simulink model "LCL_singlephase_ESO_UIO"  (R2023b)
settings: Solver=FixedStepAuto  StartTime=0.0  StopTime=0.4  FixedStep=step_time  RelTol=1e-3  EnableMultiTasking=on
values from neighbouring files (symbols this model uses):
  A = [-(rt+Rf)/Lt -1/Lt Rf/Lt ... (first row only)    [ss_LCL.m]
  Ares = [0 1; -wn^2 -2*xi*w0]    [ss_LCL.m]
  B = [Vcc/(2*Lt) ... (first row only)    [ss_LCL.m]
  Cf = 50e-6    (= 5e-05)    [ss_LCL.m]
  K = -place(Aa,Ba,p)    [ss_LCL.m]
  L = lqr(Ae,Be,blkdiag(1e5,1e5,1e5,1e5,1e5),1e-6)'    [ss_LCL.m]
  Lg = 0.1e-3    (= 0.0001)    [ss_LCL.m]
  Lt = 1e-3    (= 0.001)    [ss_LCL.m]
  rg = 0.01*0    (= 0)    [ss_LCL.m]
  rt = 0.01*0    (= 0)    [ss_LCL.m]
  step_time = 5e-7    (= 5e-07)    [ss_LCL.m]
  Vcc = 400    [ss_LCL.m]
  Vpac = 180    [ss_LCL.m]
  w0 = wn*0.01    (= 3.76991118431)    [ss_LCL.m]
  wn = 2*pi*60    (= 376.991118431)    [ss_LCL.m]
  xi = 1.0    (= 1)    [ss_LCL.m]
undefined symbols (not defined in the file or in its folder): Cfilt3, F, H, Kuio_final, Lfilt, Rfilt3, T
libraries: spsCurrentMeasurementLib x6, spsSeriesRLCBranchLib x4, spsVoltageMeasurementLib x3, spsDCVoltageSourceLib x2, spsMosfetLib x2, spsACVoltageSourceLib x1, simulink x1, spsGroundLib x1, spsTriangleGeneratorLib x1, sps_lib x1
settings Model: ExtModeTrigDuration=8  Creator=The MathWorks, Inc.  LastModifiedBy=Gustavo
settings SolverCC: AutoInsertRateTranBlk=on  MaxZcPerStep=1
settings OptimizationCC: DefaultUnderspecifiedDataType=single  EnhancedBackFolding=on  PassReuseOutputArgsAs=Individual arguments  MaxStackSize=1024  OptimizeBlockOrder=speed  DifferentSizesBufferReuse=on  OptimizationCustomize=off  DenormalBehavior=FlushToZero  EfficientTunableParamExpr=on
settings DebuggingCC: MultiTaskDSMMsg=none  ParameterPrecisionLossMsg=none  ParameterTunabilityLossMsg=error
settings HardwareCC: ProdBitPerChar=16  ProdBitPerInt=16  ProdBitPerPointer=32  ProdBitPerSizeT=32  ProdBitPerPtrDiffT=32  ProdLargestAtomicInteger=Integer  ProdLargestAtomicFloat=None  ProdWordSize=16  ProdLongLongMode=on  ProdHWDeviceType=Texas Instruments->C2000
settings ModelReferenceCC: EnableRefExpFcnMdlSchedulingChecks=on
settings SFSimCC: MATLABDynamicMemAlloc=off
settings RTWCC: Description=Embedded Coder  SystemTargetFile=ert.tlc  HardwareBoard=TI Delfino F28379D LaunchPad  TemplateMakefile=ert_default_tmf  Toolchain=Texas Instruments Code Composer Studio (C2000)  BuildConfiguration=Faster Runs  DLArmComputeVersion=19.05
settings CodeAppCC: ForceParamTrailComments=on  IgnoreCustomStorageClasses=off  OperatorAnnotations=on  SimulinkDataObjDesc=on  SFDataObjDesc=on  InsertBlockDesc=on
settings ERTTargetCC: CodeReplacementLibrary=TI C28x  ExtModeTransport=4  ExtModeStaticAlloc=on  ExtModeMexFile=ext_xcp  ExtModeIntrfLevel=Level2 - Open

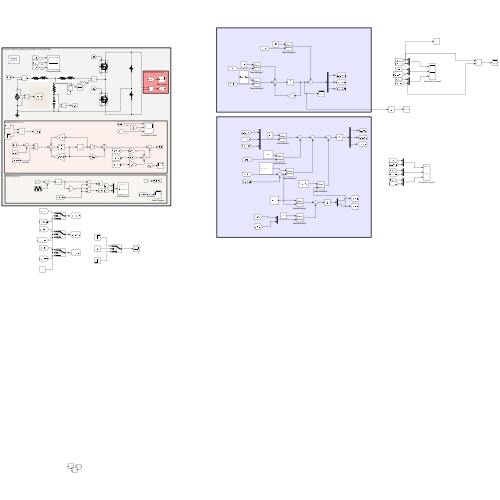
[thumbnail: Simulink's stored preview of the top-level diagram]
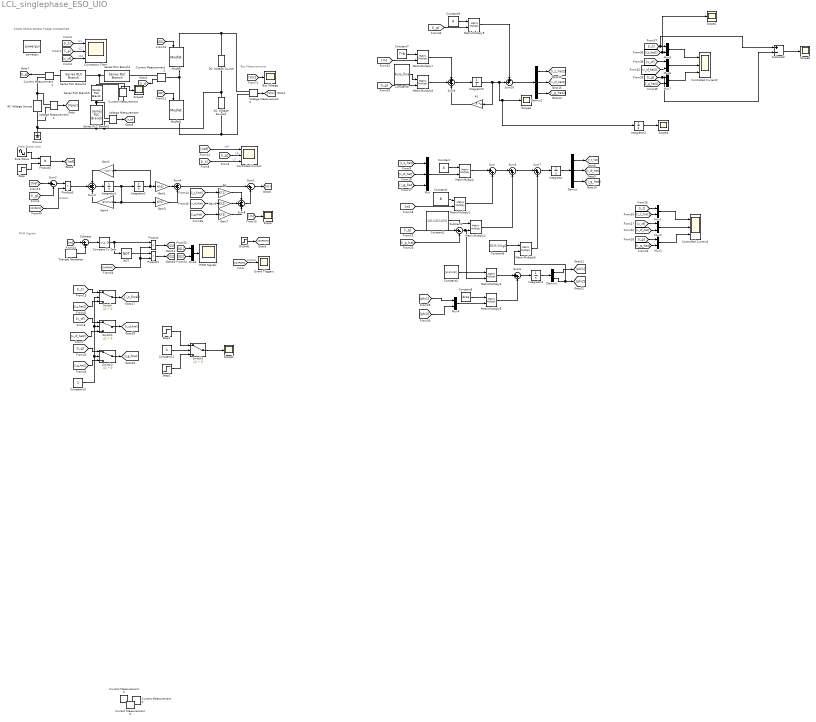
== system LCL_singlephase_ESO_UIO ==
  note: STATE SPACE SINGLE PHASE CONVERTER
  note: PWM Signals
  note: Bus Measurements
  note: State Space Loop
  A1 : Gain  Gain=F  Multiplication=Matrix(K*u) (u vector)
  A2 : Gain  Gain=K(1)
  AC Voltage Source : spsACVoltageSourceLib/AC Voltage Source  Amplitude=Vpac  Phase=90  Frequency=60  SampleTime=0  Measurements=None  BusType=swing  Pref=10e3  Qref=0  Qmin=-inf  Qmax=+inf
  Bus Voltage : Scope
  Compare To Zero : simulink/Logic and Bit Operations/Compare To Zero  relop=>=  OutDataTypeStr=boolean
  Connection Filter : Scope  NumInputPorts=3
  Constant : Constant  Value=A
  Constant1 : Constant  Value=B
  Constant10 : Constant
  Constant12 : Constant  Value=0
  Constant2 : Constant  Value=[L(1);L(2);L(3)]
  Constant4 : Constant  Value=[L(4);L(5)]
  Constant5 : Constant  Value=Ares
  Constant6 : Constant  Value=[0;0;-1/Lg]
  Constant7 : Constant  Value=T*B
  Constant8 : Constant  Value=Kuio_final
  Constant9 : Constant  Value=H
  Controlled Current : Scope  NumInputPorts=3
  Controlled Current1 : Scope  NumInputPorts=3
  Controlled Current2 : Scope  NumInputPorts=3
  Current Measurement{,1..5} (6 alike) : spsCurrentMeasurementLib/Current Measurement  PhasorSimulation=off  OutputType=Complex  PSBequivalent=0
  DC Voltage Source : spsDCVoltageSourceLib/DC Voltage Source  Amplitude=Vcc*0.5  Measurements=None
  DC Voltage Source1 : spsDCVoltageSourceLib/DC Voltage Source  Amplitude=Vcc*0.5  Measurements=None
  Demux : Demux  Outputs=3
  Demux1 : Demux  Outputs=2
  Demux2 : Demux  Outputs=3
  Event Triggers : Scope
  Gain1 : Gain  Gain=K(4)
  Gain2 : Gain  Gain=-(wn)^2
  Gain3 : Gain  Gain=K(5)
  Gain4 : Gain  Gain=-2*xi*w0
  Gain6 : Gain  Gain=K(2)
  Gain7 : Gain  Gain=K(3)
  Ground : spsGroundLib/Ground  LConnTagsString=a
  Integrator{,1..4} (5 alike) : Integrator
  Integrator5 : Integrator  InitialCondition=[0 0 -10]
  MatrixMultiply{,1..2,4..9} (9 alike) : Product  Multiplication=Matrix(*)
  Mosfet : spsMosfetLib/Mosfet  Ron=0.1  Lon=0  Rd=0.01  Vfd=0  IC=0  Rs=1e5  Cs=inf  Measurements=on
  Mosfet1 : spsMosfetLib/Mosfet  Ron=0.1  Lon=0  Rd=0.01  Vfd=0  IC=0  Rs=1e5  Cs=inf  Measurements=on
  Mux : Mux  Inputs=3
  Mux{1..8} (8 alike) : Mux  Inputs=2
  NOT : Logic  Operator=NOT  IconShape=distinctive  AllPortsSameDT=off  OutDataTypeStr=boolean
  OnGrid1 : Step  Time=0.02  SampleTime=0
  PWM Signals : Scope
  Product{,1..3} (4 alike) : Product
  Scope{,1..6} (7 alike) : Scope
  Series RLC Branch1 : spsSeriesRLCBranchLib/Series RLC Branch  LConnTagsString=__new0  RConnTagsString=__new0  BranchType=RL  Resistance=rt  Inductance=Lt  SetiL0=off  InitialCurrent=0  Capacitance=1e-6  Setx0=off  InitialVoltage=0  Measurements=None
  Series RLC Branch2 : spsSeriesRLCBranchLib/Series RLC Branch  LConnTagsString=__new0  RConnTagsString=__new0  BranchType=C  Resistance=Rfilt3  Inductance=Lfilt  SetiL0=off  InitialCurrent=0  Capacitance=Cf  Setx0=off  InitialVoltage=0  Measurements=None
  Series RLC Branch3 : spsSeriesRLCBranchLib/Series RLC Branch  LConnTagsString=__new0  RConnTagsString=__new0  BranchType=RL  Resistance=rg  Inductance=Lg  SetiL0=off  InitialCurrent=0  Capacitance=1e-6  Setx0=off  InitialVoltage=0  Measurements=None
  Series RLC Branch5 : spsSeriesRLCBranchLib/Series RLC Branch  LConnTagsString=__new0  RConnTagsString=__new0  BranchType=R  Resistance=1e-9 + 0  Inductance=Lfilt  SetiL0=off  InitialCurrent=0  Capacitance=Cfilt3  Setx0=off  InitialVoltage=0  Measurements=None
  Sine Wave : Sin  Amplitude=20  Frequency=377  SampleTime=0
  Step : Step  Time=0.1  SampleTime=0
  Step1 : Step  Time=0  SampleTime=0
  Step2 : Step  Time=0  After=0  SampleTime=0
  Subtract : Sum  Inputs=|+-
  Subtract1 : Sum  Inputs=|+-
  Subtract2 : Sum  Inputs=+-
  Sum{,1,5..7} (5 alike) : Sum  Inputs=|++
  Sum10 : Sum  Inputs=++|
  Sum2 : Sum  Inputs=|+-
  Sum{3..4,8..9} (4 alike) : Sum  Inputs=+++
  Switch{,1..3} (4 alike) : Switch  Criteria=u2 > Threshold  SaturateOnIntegerOverflow=off  InputSameDT=off
  Triangle Generator : spsTriangleGeneratorLib/Triangle Generator  Freq=20e3  Phase=0  Ts=0
  Voltage Measurement : spsVoltageMeasurementLib/Voltage Measurement  PhasorSimulation=off  OutputType=Complex  PSBequivalent=0
  Voltage Measurement1 : spsVoltageMeasurementLib/Voltage Measurement  PhasorSimulation=off  OutputType=Complex  PSBequivalent=0
  Voltage Measurement2 : spsVoltageMeasurementLib/Voltage Measurement  PhasorSimulation=off  OutputType=Complex  PSBequivalent=0
  powergui : sps_lib/powergui  Priority=1  SimulationMode=Discrete  SampleTime=step_time  frequency=60  Iterations=50  frequencyindice=60  Pbase=100e6  ErrMax=1e-4  UnitsV=kV  UnitsW=MW  buscounter=0  FunctionMessages=off  echomessages=off  EnableUseOfTLC=off  CurrentSourceSwitches=off  DisableSnubberDevices=off  DisableRonSwitches=off  DisableVfSwitches=off  DisplayEquations=off  AutomaticDiscreteSolvers=off  SolverType=Tustin/Backward Euler (TBE)  Interpol=off  ExternalGateDelay=off  methode=off  Ts=100  x0status=blocks  SPID=on  SwTol=0  HookPort=off  NonlinearTolerance=1e-4  nMaxIteration=100  ContinueOnMaxIteration=off  RestoreLinks=warning  ResistiveCurrentMeasurement=off  Frange=[0:2:500]  Ylog=off  Xlog=on  ShowGrid=off  save=off  variable=ZData  structure=0  ZoomFFT=off  StartTime=0.0  cycles=1  DisplayStyle=1  fundamental=60  FreqAxis=off  MaxFrequency=1000  frequencyindicesteady=1  RmsSteady=1  display=off
  wires:
  [Q2] -> Mosfet1/1
  [Q1] -> Mosfet/1
  Product/1 -> [Q1]
  Triangle Generator/1 -> Subtract/2
  [Q2] -> Mux8/2
  Compare To Zero/1 -> Product/1, NOT/1
  NOT/1 -> Product1/1
  Mux8/1 -> PWM Signals/1
  Subtract/1 -> Compare To Zero/1
  [Q1] -> Mux8/1
  Product1/1 -> [Q2]
  [m] -> Subtract/1
  [OnPWM] -> Product/2, Product1/2
  OnGrid1/1 -> [OnPWM]
  [i_g] -> Connection Filter/2  "IL2"
  [i_t] -> Connection Filter/1  "IL1"
  Current Measurement1/1 -> [i_g]
  Voltage Measurement/1 -> [v_cf]
  Voltage Measurement2/1 -> [Vcc]
  [Vcc] -> Bus Voltage/1
  [OnPWM] -> Event Triggers/1  "OnPWM"
  Current Measurement2/1 -> [i_t]
  [v_cf] -> Connection Filter/3  "VC3"
  [Iref] -> Sum2/1
  Gain1/1 -> Sum4/2
  Gain3/1 -> Sum4/3
  Integrator1/1 -> Gain4/1, Gain3/1, Integrator2/1
  Integrator2/1 -> Gain2/1, Gain1/1
  Gain2/1 -> Sum3/1
  Sum3/1 -> Integrator1/1
  Product3/1 -> Sum3/2
  Product2/1 -> [Iref]
  Gain7/1 -> Sum8/3
  Gain6/1 -> Sum8/2
  [i_g] -> Sum2/2
  A2/1 -> Sum8/1
  Sum4/1 -> Sum1/1
  Sum1/1 -> [m]
  Sum8/1 -> Sum1/2
  [m] -> Scope/1
  Sine Wave/1 -> Product2/1
  Step/1 -> Product2/2
  Gain4/1 -> Sum3/3
  [Iref] -> Controlled Current/1  "Iref"
  [i_g] -> Controlled Current/2  "i_g"
  [i_t] -> Controlled Current/3  "i_t"
  Voltage Measurement1/1 -> [Vpac]
  [i_t_hat] -> Mux/1
  [i_g_hat] -> Mux/3
  [v_cf_hat] -> Mux/2
  Constant/1 -> MatrixMultiply/1
  Mux/1 -> MatrixMultiply/2
  MatrixMultiply/1 -> Sum/1
  [m] -> MatrixMultiply1/2
  Constant1/1 -> MatrixMultiply1/1
  MatrixMultiply1/1 -> Sum/2
  [i_g] -> Subtract1/1
  [i_g_hat] -> Subtract1/2
  Sum/1 -> Sum5/1
  Constant2/1 -> MatrixMultiply2/1
  Subtract1/1 -> MatrixMultiply2/2, MatrixMultiply4/2
  MatrixMultiply2/1 -> Sum5/2
  Sum5/1 -> Sum7/1
  Integrator/1 -> Demux/1
  Demux/1 -> [i_t_hat]
  Demux/2 -> [v_cf_hat]
  Demux/3 -> [i_g_hat]
  Mux1/1 -> Controlled Current1/1
  Mux2/1 -> Controlled Current1/2
  Mux3/1 -> Controlled Current1/3
  [i_t_hat] -> Mux1/2
  [v_cf_hat] -> Mux2/2
  [i_g_hat] -> Mux3/2
  [i_t] -> Mux1/1
  [v_cf] -> Mux2/1
  [i_g] -> Mux3/1
  Constant4/1 -> MatrixMultiply4/1
  MatrixMultiply4/1 -> Sum6/1
  Constant5/1 -> MatrixMultiply5/1
  Mux4/1 -> MatrixMultiply5/2
  [phi1] -> Mux4/1
  [phi2] -> Mux4/2
  MatrixMultiply5/1 -> Sum6/2
  Sum6/1 -> Integrator4/1
  Demux1/1 -> [phi1]
  Sum7/1 -> Integrator/1
  MatrixMultiply6/1 -> Sum7/2
  Constant6/1 -> MatrixMultiply6/1
  Integrator4/1 -> Demux1/1
  Demux1/2 -> MatrixMultiply6/2, [phi2]
  Constant7/1 -> MatrixMultiply7/1
  [m] -> MatrixMultiply7/2
  MatrixMultiply7/1 -> Sum9/1
  Constant8/1 -> MatrixMultiply8/1
  [i_g] -> MatrixMultiply8/2
  MatrixMultiply8/1 -> Sum9/2
  Sum9/1 -> Integrator5/1
  Integrator5/1 -> Integrator3/1, Scope3/1, Sum10/2, A1/1
  A1/1 -> Sum9/3
  [i_g] -> MatrixMultiply9/2
  Constant9/1 -> MatrixMultiply9/1
  MatrixMultiply9/1 -> Sum10/1
  Demux2/2 -> [v_cf_hat2]
  Sum10/1 -> Demux2/1
  Demux2/3 -> [i_g_hat2]
  Demux2/1 -> [i_t_hat2]
  [i_t] -> Subtract2/1, Mux5/1
  Mux6/1 -> Controlled Current2/2
  Mux7/1 -> Controlled Current2/3
  [i_t_hat2] -> Scope2/1, Mux5/2
  [v_cf_hat2] -> Mux6/2
  [v_cf] -> Mux6/1
  [i_g] -> Subtract2/2, Mux7/1
  [i_g_hat2] -> Mux7/2
  Sum2/1 -> Product3/1
  [OnPWM] -> Product3/2  "OnPWM"
  [i_t] -> Switch/1
  [i_t_hat2] -> Switch/3
  [v_cf_hat2] -> Switch1/3
  [v_cf] -> Switch1/1
  [i_g_hat2] -> Switch2/3
  [i_g] -> Switch2/1
  Constant10/1 -> Switch/2, Switch1/2, Switch2/2
  Switch/1 -> [i_t_final]
  Switch1/1 -> [v_cf_final]
  Switch2/1 -> [i_g_final]
  [i_t_final] -> A2/1
  [v_cf_final] -> Gain6/1
  [i_g_final] -> Gain7/1
  Step1/1 -> Switch3/1
  Step2/1 -> Switch3/3
  Constant12/1 -> Switch3/2
  Switch3/1 -> Scope1/1
  Integrator3/1 -> Scope4/1
  Mux5/1 -> Controlled Current2/1
  Current Measurement/1 -> Scope5/1
  Subtract2/1 -> Scope6/1
  connections:
  Current Measurement2/LConn1 -- Mosfet1/LConn1 -- Mosfet/RConn1
  Current Measurement1/LConn1 -- Series RLC Branch3/LConn1
  Current Measurement1/RConn1 -- AC Voltage Source/RConn1 -- Voltage Measurement1/LConn1
  Voltage Measurement2/LConn1 -- Mosfet/LConn1 -- DC Voltage Source/RConn1
  Voltage Measurement2/LConn2 -- Mosfet1/RConn1 -- DC Voltage Source1/LConn1
  Series RLC Branch1/LConn1 -- Current Measurement/RConn1 -- Series RLC Branch3/RConn1
  Current Measurement2/RConn1 -- Series RLC Branch1/RConn1
  Voltage Measurement/LConn1 -- Series RLC Branch5/RConn1 -- Series RLC Branch2/LConn1
  Voltage Measurement/LConn2 -- Voltage Measurement1/LConn2 -- AC Voltage Source/LConn1 -- Ground/LConn1 -- Series RLC Branch2/RConn1 -- DC Voltage Source/LConn1 -- DC Voltage Source1/RConn1
  Current Measurement/LConn1 -- Series RLC Branch5/LConn1
